simulink subsystem "HMT"  (R2022b)
settings: Solver=VariableStepAuto  StartTime=0.0  StopTime=10.0  RelTol=1e-3
libraries: fl_lib x21, nesl_utility x17, sh_lib x8, sdl_lib x4
settings Model: Creator=david  LastModifiedBy=david

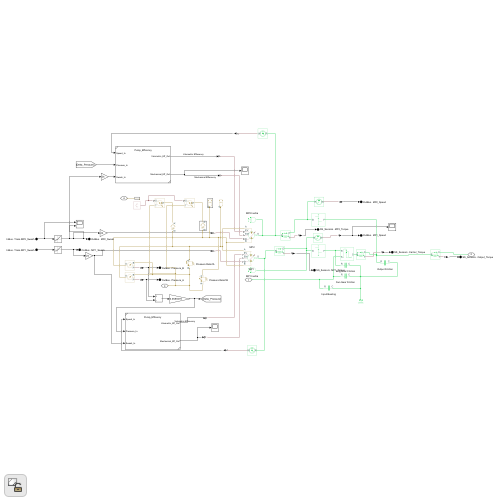
[thumbnail: Simulink's stored preview of the top-level diagram]
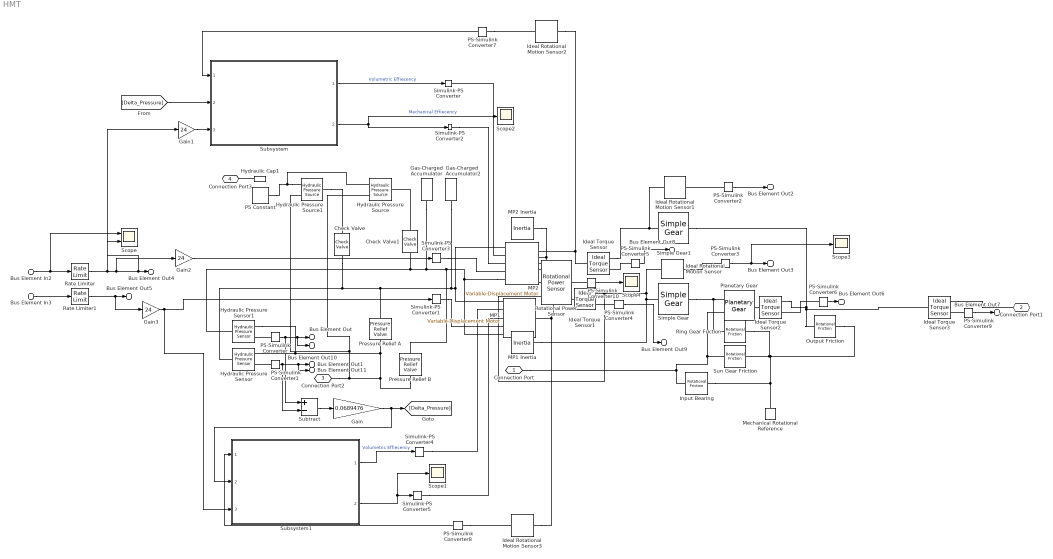
== system HMT ==
  Bus Element In3 : Inport  PortName=InBus  Element=MP1_Swash
  Bus Element In2 : Inport  PortName=InBus  Element=MP2_Swash
  Check Valve : sh_lib/Valves/Directional Valves/Check Valve  area_max=1e-4 m^2  pres_crack=0.3e5 Pa  pres_max=1.2e5 Pa  C_d=0.7  A_leak=.001 in^2  lam_spec=1  B_lam=0.999  Re_cr=12  dynamic=0  tau=0.1 s  area_init=1e-12 m^2
      settings: InternalSimscapePortConfiguration="{\"Bottom\":[],\"Left\":[{\"id\":\"A\",\"label\":\"A\",\"type\":\"foundation.hydraulic.hydraulic\"}],\"Right\":[{\"id\":\"B\",\"label\":\"B\",\"type\":\"foundation.hydraulic.hydraulic\"}],\"Top\":[]}"
  Check Valve1 : sh_lib/Valves/Directional Valves/Check Valve  area_max=1e-4 m^2  pres_crack=0.3e5 Pa  pres_max=1.2e5 Pa  C_d=0.7  A_leak=.001 in^2  lam_spec=1  B_lam=0.999  Re_cr=12  dynamic=0  tau=0.1 s  area_init=1e-12 m^2
      settings: InternalSimscapePortConfiguration="{\"Bottom\":[],\"Left\":[{\"id\":\"A\",\"label\":\"A\",\"type\":\"foundation.hydraulic.hydraulic\"}],\"Right\":[{\"id\":\"B\",\"label\":\"B\",\"type\":\"foundation.hydraulic.hydraulic\"}],\"Top\":[]}"
  Gain : Gain  Gain=0.0689476
  Gain1 : Gain  Gain=24
  Gain2 : Gain  Gain=24
  Gain3 : Gain  Gain=24
  Gas-Charged Accumulator : sh_lib/Accumulators/Gas-Charged Accumulator  capacity=2 in^3  dead_volume=1 in^3  pr_preload=2000 psi  k_sh=1.4  stiff_coeff=1e10 Pa/m^3  penetr_coeff=1e10 Pa*s/m^6  flow_rate_specify=off  flow_rate_priority=None  flow_rate=5e-3 m^3/s  flow_rate_nominal_specify=off  flow_rate_nominal_unit=m^3/s  flow_rate_nominal_value=1  liquid_volume_specify=on  liquid_volume_priority=High  liquid_volume=1 in^3  liquid_volume_nominal_specify=off  liquid_volume_nominal_unit=m^3  liquid_volume_nominal_value=1  liquid_pressure_specify=off  liquid_pressure_priority=None  liquid_pressure=1.01325e5 Pa  liquid_pressure_nominal_specify=off  liquid_pressure_nominal_unit=Pa  liquid_pressure_nominal_value=1
      settings: InternalSimscapePortConfiguration="{\"Bottom\":[],\"Left\":[],\"Right\":[{\"id\":\"A\",\"label\":\"A\",\"type\":\"foundation.hydraulic.hydraulic\"}],\"Top\":[]}"
  Gas-Charged Accumulator2 : sh_lib/Accumulators/Gas-Charged Accumulator  capacity=2 in^3  dead_volume=1 in^3  pr_preload=2000 psi  k_sh=1.4  stiff_coeff=1e10 Pa/m^3  penetr_coeff=1e10 Pa*s/m^6  flow_rate_specify=off  flow_rate_priority=None  flow_rate=5e-3 m^3/s  flow_rate_nominal_specify=off  flow_rate_nominal_unit=m^3/s  flow_rate_nominal_value=1  liquid_volume_specify=on  liquid_volume_priority=High  liquid_volume=1 in^3  liquid_volume_nominal_specify=off  liquid_volume_nominal_unit=m^3  liquid_volume_nominal_value=1  liquid_pressure_specify=off  liquid_pressure_priority=None  liquid_pressure=1.01325e5 Pa  liquid_pressure_nominal_specify=off  liquid_pressure_nominal_unit=Pa  liquid_pressure_nominal_value=1
      settings: InternalSimscapePortConfiguration="{\"Bottom\":[],\"Left\":[],\"Right\":[{\"id\":\"A\",\"label\":\"A\",\"type\":\"foundation.hydraulic.hydraulic\"}],\"Top\":[]}"
  Hydraulic Cap1 : fl_lib/Hydraulic/Hydraulic Elements/Hydraulic Cap  p_specify=off  p_priority=None  p=0 Pa  p_nominal_specify=off  p_nominal_unit=Pa  p_nominal_value=1
      settings: InternalSimscapePortConfiguration="{\"Bottom\":[],\"Left\":[{\"id\":\"P\",\"label\":\"\",\"type\":\"foundation.hydraulic.hydraulic\"}],\"Right\":[],\"Top\":[]}"
  Hydraulic Pressure Sensor : fl_lib/Hydraulic/Hydraulic Sensors/Hydraulic Pressure Sensor
  Hydraulic Pressure Sensor1 : fl_lib/Hydraulic/Hydraulic Sensors/Hydraulic Pressure Sensor
  Hydraulic Pressure Source : fl_lib/Hydraulic/Hydraulic Sources/Hydraulic Pressure Source
      settings: InternalSimscapePortConfiguration="{\"Bottom\":[],\"Left\":[{\"id\":\"P\",\"label\":\"P\",\"type\":\"foundation.hydraulic.hydraulic\"}],\"Right\":[{\"id\":\"S\",\"label\":\"S\",\"type\":\"input\"},{\"id\":\"T\",\"label\":\"T\",\"type\":\"foundation.hydraulic.hydraulic\"}],\"Top\":[]}"
  Hydraulic Pressure Source1 : fl_lib/Hydraulic/Hydraulic Sources/Hydraulic Pressure Source
      settings: InternalSimscapePortConfiguration="{\"Bottom\":[],\"Left\":[{\"id\":\"P\",\"label\":\"P\",\"type\":\"foundation.hydraulic.hydraulic\"}],\"Right\":[{\"id\":\"S\",\"label\":\"S\",\"type\":\"input\"},{\"id\":\"T\",\"label\":\"T\",\"type\":\"foundation.hydraulic.hydraulic\"}],\"Top\":[]}"
  Ideal Rotational Motion Sensor{,1..3} (4 alike) : fl_lib/Mechanical/Mechanical Sensors/Ideal Rotational Motion Sensor  reference=foundation.enum.MeasurementReference.absolute  acceleration_port=false  velocity_port=true  position_port=false  wrap_angle=false  offset=0 rad
      settings: InternalSimscapePortConfiguration="{\"Bottom\":[],\"Left\":[{\"id\":\"R\",\"label\":\"R\",\"type\":\"foundation.mechanical.rotational.rotational\"}],\"Right\":[{\"id\":\"W\",\"label\":\"W\",\"type\":\"output\"}],\"Top\":[]}"
  Ideal Torque Sensor{,1..3} (4 alike) : fl_lib/Mechanical/Mechanical Sensors/Ideal Torque Sensor
  Input Bearing : fl_lib/Mechanical/Rotational Elements/Rotational Friction  brkwy_trq=1 lbf*ft  brkwy_vel=0.1 rad/s  Col_trq=.5 lbf*ft  visc_coef=0.001 N*m*s/rad  w_specify=off  w_priority=None  w=0 rad/s  w_nominal_specify=off  w_nominal_unit=rad/s  w_nominal_value=1  t_specify=off  t_priority=None  t=0 N*m  t_nominal_specify=off  t_nominal_unit=N*m  t_nominal_value=1
  MP1 : sh_lib/Pumps and Motors/Variable-Displacement Motor  mdl_type=2  stroke_max=1 m  D_max=24 cm^3/rev  cntrl_mem_tab=[-1,0,1] m  displ_tab=[-24,0,24] cm^3/rev  interp_method=2  extrap_method=2  loss_spec=1  w_nominal=4000 rpm  pr_nominal=2000 psi  visc_nominal=18 cSt  dens_nominal=900 kg/m^3  efficiency_vol=0.95  no_load_torque=0.05 N*m  torque_pressure_coeff=0.6e-6 N*m/Pa  p_diff_eff_TLU=[10,135,278] bar  omega_eff_TLU=[500,1974,4000] rpm  displacement_eff_TLU=[4.8,12,24] cm^3/rev  vol_eff_TLU=cat(3,[.47,0.01,0.01; .98,.38,.01;.98,.67,.38],[.81,.12,0.01;.99,.80,.65;1.00,.88,.79],[.93,.61,.42;1.00,.91,.85;1.00,.95,.89])  mech_eff_TLU=cat(3,[.46,.62,.54;.27,.74,.83;.21,.73,.89],[.65,.86,.83;.46,.86,.94;.35,.86,.95],[.66,.83,.85;.53,.88,.91;.39,.87,.94])  p_diff_loss_TLU=[100000, 1000000, 2000000] Pa  omega_loss_TLU=[25, 50, 100, 200, 300, 400] rad/s  displacement_loss_TLU=[-30, -19, 19, 30] cm^3/rev  vol_loss_TLU=repmat([.0282, .0253, .0241, .0235, .0291, .0325; .2596, .1271, .1017, .0917, .1216, .1142; .7874, .1901, .141, .1211, .1797, .1978] * 1e-3, 1, 1, 4) m^3/s  mech_loss_TLU=repmat([.002, .002, .002, .002, .002, .002; .06, .055, .055, .055, .055, .05; .19, .19, .18, .18, .17, .16], 1, 1, 4) N*m  pressure_threshold=10 psi  omega_threshold=10 rad/s  displacement_threshold=0.5 cm^3/rev  octant_check=0  pressure_check=0  min_valid_pressure=0 Pa  vol_eff_min=1  vol_eff_max=1  mech_eff_min=.01  mech_eff_max=1
      settings: InternalSimscapePortConfiguration="{\"Bottom\":[],\"Left\":[{\"id\":\"A\",\"label\":\"A\",\"type\":\"foundation.hydraulic.hydraulic\"},{\"id\":\"EV\",\"label\":\"EV\",\"type\":\"input\"},{\"id\":\"EM\",\"label\":\"EM\",\"type\":\"input\"},{\"id\":\"D\",\"label\":\"D\",\"type\":\"input\"},{\"id\":\"B\",\"label\":\"B\",\"type\":\"foundation.hydraulic.hydraulic\"}],\"Right\":[{\"id\":\"S\",\"label\":\"S\",\"type\":\"foundation.mechanical.rotational.rotational\"}],\"Top\":[]}"
  MP1 Inertia : fl_lib/Mechanical/Rotational Elements/Inertia  inertia=0.0009 kg*m^2  num_ports=foundation.enum.numPorts2.one  w_specify=off  w_priority=Low  w=0 rad/s  w_nominal_specify=off  w_nominal_unit=rad/s  w_nominal_value=1  t_specify=off  t_priority=None  t=0 N*m  t_nominal_specify=off  t_nominal_unit=N*m  t_nominal_value=1
  MP2 : sh_lib/Pumps and Motors/Variable-Displacement Motor  mdl_type=2  stroke_max=1 m  D_max=24 cm^3/rev  cntrl_mem_tab=[-1,0,1] m  displ_tab=[-24,0,24] cm^3/rev  interp_method=2  extrap_method=2  loss_spec=1  w_nominal=4000 rpm  pr_nominal=2000 psi  visc_nominal=18 cSt  dens_nominal=900 kg/m^3  efficiency_vol=0.95  no_load_torque=0.05 N*m  torque_pressure_coeff=0.6e-6 N*m/Pa  p_diff_eff_TLU=[10,135,278] bar  omega_eff_TLU=[500,1974,4000] rpm  displacement_eff_TLU=[4.8,12,24] cm^3/rev  vol_eff_TLU=cat(3,[.47,0.01,0.01; .98,.38,.01;.98,.67,.38],[.81,.12,0.01;.99,.80,.65;1.00,.88,.79],[.93,.61,.42;1.00,.91,.85;1.00,.95,.89])  mech_eff_TLU=cat(3,[.46,.62,.54;.27,.74,.83;.21,.73,.89],[.65,.86,.83;.46,.86,.94;.35,.86,.95],[.66,.83,.85;.53,.88,.91;.39,.87,.94])  p_diff_loss_TLU=[100000, 1000000, 2000000] Pa  omega_loss_TLU=[25, 50, 100, 200, 300, 400] rad/s  displacement_loss_TLU=[-30, -19, 19, 30] cm^3/rev  vol_loss_TLU=repmat([.0282, .0253, .0241, .0235, .0291, .0325; .2596, .1271, .1017, .0917, .1216, .1142; .7874, .1901, .141, .1211, .1797, .1978] * 1e-3, 1, 1, 4) m^3/s  mech_loss_TLU=repmat([.002, .002, .002, .002, .002, .002; .06, .055, .055, .055, .055, .05; .19, .19, .18, .18, .17, .16], 1, 1, 4) N*m  pressure_threshold=10 psi  omega_threshold=10 rad/s  displacement_threshold=0.5 cm^3/rev  octant_check=0  pressure_check=0  min_valid_pressure=0 Pa  vol_eff_min=.01  vol_eff_max=1  mech_eff_min=.01  mech_eff_max=1
      settings: InternalSimscapePortConfiguration="{\"Bottom\":[],\"Left\":[{\"id\":\"A\",\"label\":\"A\",\"type\":\"foundation.hydraulic.hydraulic\"},{\"id\":\"EV\",\"label\":\"EV\",\"type\":\"input\"},{\"id\":\"EM\",\"label\":\"EM\",\"type\":\"input\"},{\"id\":\"D\",\"label\":\"D\",\"type\":\"input\"},{\"id\":\"B\",\"label\":\"B\",\"type\":\"foundation.hydraulic.hydraulic\"}],\"Right\":[{\"id\":\"S\",\"label\":\"S\",\"type\":\"foundation.mechanical.rotational.rotational\"}],\"Top\":[]}"
  MP2 Inertia : fl_lib/Mechanical/Rotational Elements/Inertia  inertia=0.0009 kg*m^2  num_ports=foundation.enum.numPorts2.one  w_specify=on  w_priority=Low  w=0 rpm  w_nominal_specify=off  w_nominal_unit=rad/s  w_nominal_value=1  t_specify=off  t_priority=None  t=0 N*m  t_nominal_specify=off  t_nominal_unit=N*m  t_nominal_value=1
  Mechanical Rotational Reference : fl_lib/Mechanical/Rotational Elements/Mechanical Rotational Reference
  Output Friction : fl_lib/Mechanical/Rotational Elements/Rotational Friction  brkwy_trq=1 lbf*ft  brkwy_vel=0.1 rad/s  Col_trq=.5 lbf*ft  visc_coef=0.001 N*m*s/rad  w_specify=off  w_priority=None  w=0 rad/s  w_nominal_specify=off  w_nominal_unit=rad/s  w_nominal_value=1  t_specify=off  t_priority=None  t=0 N*m  t_nominal_specify=off  t_nominal_unit=N*m  t_nominal_value=1
  PS Constant : fl_lib/Physical Signals/Sources/PS Constant  constant=100 psi
  PS-Simulink Converter : nesl_utility/PS-Simulink Converter  PhysicalDomain=network_engine_domain  SubClassName=ps_output  LeftPortType=input  RightPortType=output  PseudoPeriodic=off  Frequencies=[]  VectorFormat=inherit  Unit=psi  AffineConversion=off
  PS-Simulink Converter1 : nesl_utility/PS-Simulink Converter  PhysicalDomain=network_engine_domain  SubClassName=ps_output  LeftPortType=input  RightPortType=output  PseudoPeriodic=off  Frequencies=[]  VectorFormat=inherit  Unit=psi  AffineConversion=off
  PS-Simulink Converter10 : nesl_utility/PS-Simulink Converter  PhysicalDomain=network_engine_domain  SubClassName=ps_output  LeftPortType=input  RightPortType=output  PseudoPeriodic=off  Frequencies=[]  VectorFormat=inherit  Unit=inherit  AffineConversion=off
  PS-Simulink Converter{2..3,7..8} (4 alike) : nesl_utility/PS-Simulink Converter  PhysicalDomain=network_engine_domain  SubClassName=ps_output  LeftPortType=input  RightPortType=output  PseudoPeriodic=off  Frequencies=[]  VectorFormat=inherit  Unit=rpm  AffineConversion=off
  PS-Simulink Converter4 : nesl_utility/PS-Simulink Converter  PhysicalDomain=network_engine_domain  SubClassName=ps_output  LeftPortType=input  RightPortType=output  PseudoPeriodic=off  Frequencies=[]  VectorFormat=inherit  Unit=in*lb  AffineConversion=off
  PS-Simulink Converter5 : nesl_utility/PS-Simulink Converter  PhysicalDomain=network_engine_domain  SubClassName=ps_output  LeftPortType=input  RightPortType=output  PseudoPeriodic=off  Frequencies=[]  VectorFormat=inherit  Unit=in*lb  AffineConversion=off
  PS-Simulink Converter6 : nesl_utility/PS-Simulink Converter  PhysicalDomain=network_engine_domain  SubClassName=ps_output  LeftPortType=input  RightPortType=output  PseudoPeriodic=off  Frequencies=[]  VectorFormat=inherit  Unit=ft*lb  AffineConversion=off
  PS-Simulink Converter9 : nesl_utility/PS-Simulink Converter  PhysicalDomain=network_engine_domain  SubClassName=ps_output  LeftPortType=input  RightPortType=output  PseudoPeriodic=off  Frequencies=[]  VectorFormat=inherit  Unit=ft*lb  AffineConversion=off
  Planetary Gear : sdl_lib/Gears/Planetary Gear  rs_ratio=2.636  friction_model=sdl.enum.gear_friction.constant  efficiency=[.96, .98]  temperature_TLU=[280, 300, 320] K  efficiency_sp_TLU=[.95, .9, .85]  efficiency_rp_TLU=[.95, .9, .85]  pwr_thr=[.001, .001] W  mu_visc=[0, 0] N*m*s/rad  model_inertia=simscape.enum.onoff.off  planet_inertia=0.001 kg*m^2  thermal_mass=50 J/K  T_init=300 K
  Pressure Relief A : sh_lib/Valves/Pressure Control Valves/Pressure Relief Valve  valve_area_spec=1  p_diff_TLU=[30.15e5 : 15e3 : 31.35e5] Pa  area_TLU=[1 : 1 : 9] .* 1e-5 m^2  area_max=1e-4 m^2  pres_set=4000 psi  reg_range=5e5 Pa  C_d=0.7  A_leak=1e-12 m^2  lam_spec=1  B_lam=0.999  Re_cr=12  dynamic=0  tau=0.1 s  area_init=1e-12 m^2
      settings: InternalSimscapePortConfiguration="{\"Bottom\":[],\"Left\":[{\"id\":\"A\",\"label\":\"A\",\"type\":\"foundation.hydraulic.hydraulic\"}],\"Right\":[{\"id\":\"B\",\"label\":\"B\",\"type\":\"foundation.hydraulic.hydraulic\"}],\"Top\":[]}"
  Pressure Relief B : sh_lib/Valves/Pressure Control Valves/Pressure Relief Valve  valve_area_spec=1  p_diff_TLU=[30.15e5 : 15e3 : 31.35e5] Pa  area_TLU=[1 : 1 : 9] .* 1e-5 m^2  area_max=1e-4 m^2  pres_set=4000 psi  reg_range=5e5 Pa  C_d=0.7  A_leak=1e-12 m^2  lam_spec=1  B_lam=0.999  Re_cr=12  dynamic=0  tau=0.1 s  area_init=1e-12 m^2
      settings: InternalSimscapePortConfiguration="{\"Bottom\":[],\"Left\":[{\"id\":\"A\",\"label\":\"A\",\"type\":\"foundation.hydraulic.hydraulic\"}],\"Right\":[{\"id\":\"B\",\"label\":\"B\",\"type\":\"foundation.hydraulic.hydraulic\"}],\"Top\":[]}"
  Rate Limiter : RateLimiter  RisingSlewLimit=.5  FallingSlewLimit=-.5  SampleTimeMode=inherited
  Rate Limiter1 : RateLimiter  RisingSlewLimit=.5  FallingSlewLimit=-.5  SampleTimeMode=inherited
  Ring Gear Friction : fl_lib/Mechanical/Rotational Elements/Rotational Friction  brkwy_trq=1 lbf*ft  brkwy_vel=0.1 rad/s  Col_trq=.5 lbf*ft  visc_coef=0.001 N*m*s/rad  w_specify=off  w_priority=None  w=0 rad/s  w_nominal_specify=off  w_nominal_unit=rad/s  w_nominal_value=1  t_specify=off  t_priority=None  t=0 N*m  t_nominal_specify=off  t_nominal_unit=N*m  t_nominal_value=1
  Rotational Power Sensor : sdl_lib/Sensors/Rotational Power Sensor  measurement_type=sdl.enum.rotationalPowerSensorType.instantaneous  averaging_period=1 s  max_frequency=1000 Hz  max_speed=1000 rpm
      settings: InternalSimscapePortConfiguration="{\"Bottom\":[],\"Left\":[{\"id\":\"S\",\"label\":\"S\",\"type\":\"foundation.mechanical.rotational.rotational\"},{\"id\":\"R\",\"label\":\"R\",\"type\":\"foundation.mechanical.rotational.rotational\"},{\"id\":\"C\",\"label\":\"C\",\"type\":\"foundation.mechanical.rotational.rotational\"}],\"Right\":[{\"id\":\"P\",\"label\":\"P\",\"type\":\"output\"}],\"Top\":[]}"
  Scope : Scope  NumInputPorts=2
  Scope{1..4} (4 alike) : Scope
  Simple Gear : sdl_lib/Gears/Simple Gear  ratio=2.16  rotation_direction=sdl.enum.shaftOutputDirection.opposite  friction_model=sdl.enum.gear_efficiencies_load.constant  T_noload=0.1 N*m  T_nom=5 N*m  efficiency_nom=0.8  efficiency=0.98  temperature_TLU=[280, 300, 320] K  load_TLU=[1, 5, 10] N*m  efficiency_TLU=[.95, .9, .85]  efficiency_TLU2=[.85, .8, .75; .95, .9, .85; .85, .8, .7]  w_thr=0.01 rad/s  pwr_thr=0.001 W  backlash_model=sdl.enum.backlashModel.Off  backlash_distance=1e-3 mm  x0=0 mm  r_base=0.1 m  hardstop_model=simscape.enum.hardstop.smooth  transition=1e-4 mm  backlash_stiffness=1e7 N/m  backlash_damping=1e6 N*s/m  e=0  v_tol=0.001 m/s  mu_visc=[0, 0] N*m*s/rad  enable_faults=simscape.enum.onoff.off  efficiency_fault=0.05  external_fault=simscape.enum.onoff.off  temporal_fault=simscape.enum.onoff.off  fault_time=5 s  fault_angles=pi / 12 rad  report_fault=simscape.enum.assert.action.none  thermal_mass=50 J/K  temperature_specify=off  temperature_priority=High  temperature=300 K  temperature_nominal_specify=off  temperature_nominal_unit=K  temperature_nominal_value=1  x_backlash_specify=off  x_backlash_priority=None  x_backlash=0 mm  x_backlash_nominal_specify=off  x_backlash_nominal_unit=mm  x_backlash_nominal_value=1  f_hardstop_specify=off  f_hardstop_priority=None  f_hardstop=0 N  f_hardstop_nominal_specify=off  f_hardstop_nominal_unit=N  f_hardstop_nominal_value=1  v_backlash_specify=off  v_backlash_priority=None  v_backlash=0 m/s  v_backlash_nominal_specify=off  v_backlash_nominal_unit=m/s  v_backlash_nominal_value=1
  Simple Gear1 : sdl_lib/Gears/Simple Gear  ratio=2.714  rotation_direction=sdl.enum.shaftOutputDirection.opposite  friction_model=sdl.enum.gear_efficiencies_load.constant  T_noload=0.1 N*m  T_nom=5 N*m  efficiency_nom=0.8  efficiency=0.98  temperature_TLU=[280, 300, 320] K  load_TLU=[1, 5, 10] N*m  efficiency_TLU=[.95, .9, .85]  efficiency_TLU2=[.85, .8, .75; .95, .9, .85; .85, .8, .7]  w_thr=0.01 rad/s  pwr_thr=0.001 W  backlash_model=sdl.enum.backlashModel.Off  backlash_distance=1e-3 mm  x0=0 mm  r_base=0.1 m  hardstop_model=simscape.enum.hardstop.smooth  transition=1e-4 mm  backlash_stiffness=1e7 N/m  backlash_damping=1e6 N*s/m  e=0  v_tol=0.001 m/s  mu_visc=[0, 0] N*m*s/rad  enable_faults=simscape.enum.onoff.off  efficiency_fault=0.05  external_fault=simscape.enum.onoff.off  temporal_fault=simscape.enum.onoff.off  fault_time=5 s  fault_angles=pi / 12 rad  report_fault=simscape.enum.assert.action.none  thermal_mass=50 J/K  temperature_specify=off  temperature_priority=High  temperature=300 K  temperature_nominal_specify=off  temperature_nominal_unit=K  temperature_nominal_value=1  x_backlash_specify=off  x_backlash_priority=None  x_backlash=0 mm  x_backlash_nominal_specify=off  x_backlash_nominal_unit=mm  x_backlash_nominal_value=1  f_hardstop_specify=off  f_hardstop_priority=None  f_hardstop=0 N  f_hardstop_nominal_specify=off  f_hardstop_nominal_unit=N  f_hardstop_nominal_value=1  v_backlash_specify=off  v_backlash_priority=None  v_backlash=0 m/s  v_backlash_nominal_specify=off  v_backlash_nominal_unit=m/s  v_backlash_nominal_value=1
  Simulink-PS Converter{,2,4..5} (4 alike) : nesl_utility/Simulink-PS Converter  PhysicalDomain=network_engine_domain  SubClassName=ps_input  LeftPortType=input  RightPortType=output  PseudoPeriodic=off  Frequencies=[]  NoiseDistribution=none  NoiseParameters=[]  Unit=1  AffineConversion=off  FilteringAndDerivatives=provide  SimscapeFilterOrder=1  InputFilterTimeConstant=0.001  UdotUserProvided=0
  Simulink-PS Converter1 : nesl_utility/Simulink-PS Converter  PhysicalDomain=network_engine_domain  SubClassName=ps_input  LeftPortType=input  RightPortType=output  PseudoPeriodic=off  Frequencies=[]  NoiseDistribution=none  NoiseParameters=[]  Unit=cm^3/rev  AffineConversion=off  FilteringAndDerivatives=provide  SimscapeFilterOrder=1  InputFilterTimeConstant=0.001  UdotUserProvided=0
  Simulink-PS Converter3 : nesl_utility/Simulink-PS Converter  PhysicalDomain=network_engine_domain  SubClassName=ps_input  LeftPortType=input  RightPortType=output  PseudoPeriodic=off  Frequencies=[]  NoiseDistribution=none  NoiseParameters=[]  Unit=cm^3/rev  AffineConversion=off  FilteringAndDerivatives=provide  SimscapeFilterOrder=1  InputFilterTimeConstant=0.001  UdotUserProvided=0
  Subsystem : Subsystem  ReferencedSubsystem=Pump_Efficency
  Subsystem1 : Subsystem  ReferencedSubsystem=Pump_Efficency
  Subtract : Sum  Inputs=+-
  Sun Gear Friction : fl_lib/Mechanical/Rotational Elements/Rotational Friction  brkwy_trq=1 lbf*ft  brkwy_vel=0.1 rad/s  Col_trq=.5 lbf*ft  visc_coef=0.001 N*m*s/rad  w_specify=off  w_priority=None  w=0 rad/s  w_nominal_specify=off  w_nominal_unit=rad/s  w_nominal_value=1  t_specify=off  t_priority=None  t=0 N*m  t_nominal_specify=off  t_nominal_unit=N*m  t_nominal_value=1
  Connection Port : PMIOPort  Side=Right
  Connection Port1 : PMIOPort  Port=2  Side=Left
  Connection Port2 : PMIOPort  Port=3  Side=Right
  Connection Port3 : PMIOPort  Port=4  Side=Left
  Bus Element Out : Outport  VectorParamsAs1DForOutWhenUnconnected=off  PortName=OutBus  Element=Pressure_B
  Bus Element Out1 : Outport  VectorParamsAs1DForOutWhenUnconnected=off  PortName=OutBus  Element=Pressure_A
  Bus Element Out2 : Outport  VectorParamsAs1DForOutWhenUnconnected=off  PortName=OutBus  Element=MP2_Speed
  Bus Element Out3 : Outport  VectorParamsAs1DForOutWhenUnconnected=off  PortName=OutBus  Element=MP1_Speed
  Bus Element Out4 : Outport  VectorParamsAs1DForOutWhenUnconnected=off  PortName=OutBus  Element=MP2_Swash
  Bus Element Out5 : Outport  VectorParamsAs1DForOutWhenUnconnected=off  PortName=OutBus  Element=MP1_Swash
  Bus Element Out9 : Outport  Port=2  VectorParamsAs1DForOutWhenUnconnected=off  PortName=SS_Sensors  Element=MP1_Torque
  Bus Element Out8 : Outport  Port=2  VectorParamsAs1DForOutWhenUnconnected=off  PortName=SS_Sensors  Element=MP2_Torque
  Bus Element Out6 : Outport  Port=2  VectorParamsAs1DForOutWhenUnconnected=off  PortName=SS_Sensors  Element=Carrier_Torque
  Bus Element Out7 : Outport  Port=2  VectorParamsAs1DForOutWhenUnconnected=off  PortName=SS_Sensors  Element=Output_Torque
  Bus Element Out10 : Outport  Port=2  VectorParamsAs1DForOutWhenUnconnected=off  PortName=SS_Sensors  Element=Pressure_B
  Bus Element Out11 : Outport  Port=2  VectorParamsAs1DForOutWhenUnconnected=off  PortName=SS_Sensors  Element=Pressure_A
  wires:
  PS-Simulink Converter10/1 -> Scope4/1
  PS-Simulink Converter9/1 -> Bus Element Out7/1
  Gain1/1 -> Subsystem/3
  PS-Simulink Converter7/1 -> Subsystem/1
  Bus Element In2/1 -> Rate Limiter/1, Scope/1
  Rate Limiter1/1 -> Gain3/1, Bus Element Out5/1
  Bus Element In3/1 -> Rate Limiter1/1
  PS-Simulink Converter3/1 -> Bus Element Out3/1, Scope3/1
  PS-Simulink Converter2/1 -> Bus Element Out2/1
  PS-Simulink Converter/1 -> Bus Element Out/1, Bus Element Out10/1, Subtract/1
  PS-Simulink Converter1/1 -> Bus Element Out1/1, Bus Element Out11/1, Subtract/2
  PS-Simulink Converter5/1 -> Bus Element Out8/1
  PS-Simulink Converter6/1 -> Bus Element Out6/1
  PS-Simulink Converter4/1 -> Bus Element Out9/1
  Subsystem/1 -> Simulink-PS Converter/1  "Volumetric Effiecency"
  Subsystem/2 -> Simulink-PS Converter2/1, Scope2/1  "Mechanical Effiecency"
  Subtract/1 -> Gain/1
  [Delta_Pressure] -> Subsystem/2
  Rate Limiter/1 -> Scope/2, Gain2/1, Gain1/1, Bus Element Out4/1
  Gain2/1 -> Simulink-PS Converter3/1
  Subsystem1/1 -> Simulink-PS Converter4/1  "Volumetric Effiecency"
  PS-Simulink Converter8/1 -> Subsystem1/1
  Gain3/1 -> Subsystem1/3, Simulink-PS Converter1/1
  Gain/1 -> Subsystem1/2, [Delta_Pressure]
  Subsystem1/2 -> Simulink-PS Converter5/1, Scope1/1
  connections:
  Rotational Power Sensor/LConn2 -- Ideal Rotational Motion Sensor2/LConn1 -- Ideal Torque Sensor/LConn1
  Input Bearing/RConn1 -- Ring Gear Friction/RConn1 -- Sun Gear Friction/RConn1 -- Output Friction/RConn1 -- Mechanical Rotational Reference/LConn1
  Planetary Gear/RConn1 -- Ring Gear Friction/LConn1 -- Simple Gear/RConn1
  Sun Gear Friction/LConn1 -- Connection Port/RConn1 -- Input Bearing/LConn1 -- Planetary Gear/RConn2
  Hydraulic Pressure Source1/RConn1 -- Hydraulic Pressure Source/RConn1 -- PS Constant/RConn1
  MP2/LConn5 -- Hydraulic Pressure Sensor1/LConn1 -- Check Valve1/RConn1 -- Gas-Charged Accumulator/RConn1 -- Pressure Relief B/LConn1 -- MP1/LConn5
  MP2/RConn1 -- MP2 Inertia/LConn1 -- Rotational Power Sensor/LConn1
  Ideal Torque Sensor1/RConn1 -- MP1 Inertia/LConn1 -- Simple Gear/LConn1 -- Ideal Rotational Motion Sensor/LConn1 -- Rotational Power Sensor/LConn3
  Output Friction/LConn1 -- Ideal Torque Sensor2/RConn1 -- Simple Gear1/RConn1 -- Ideal Torque Sensor3/LConn1
  Hydraulic Pressure Source1/RConn2 -- Hydraulic Pressure Sensor/RConn1 -- Hydraulic Pressure Sensor1/RConn1 -- Pressure Relief A/RConn1 -- Pressure Relief B/RConn1 -- Connection Port2/RConn1 -- Hydraulic Pressure Source/RConn2
  Hydraulic Pressure Sensor/LConn1 -- MP2/LConn1 -- MP1/LConn1 -- Gas-Charged Accumulator2/RConn1 -- Pressure Relief A/LConn1 -- Check Valve/RConn1
  Ideal Torque Sensor/RConn1 -- Simple Gear1/LConn1 -- Ideal Rotational Motion Sensor1/LConn1
  Ideal Rotational Motion Sensor3/LConn1 -- MP1/RConn1 -- Ideal Torque Sensor1/LConn1
  PS-Simulink Converter10/LConn1 -- Rotational Power Sensor/RConn1
  PS-Simulink Converter9/LConn1 -- Ideal Torque Sensor3/RConn2
  Ideal Torque Sensor3/RConn1 -- Connection Port1/RConn1
  Check Valve1/LConn1 -- Hydraulic Pressure Source/LConn1
  Hydraulic Pressure Source1/LConn1 -- Check Valve/LConn1
  Hydraulic Cap1/LConn1 -- Connection Port3/RConn1
  PS-Simulink Converter3/LConn1 -- Ideal Rotational Motion Sensor/RConn1
  PS-Simulink Converter2/LConn1 -- Ideal Rotational Motion Sensor1/RConn1
  PS-Simulink Converter1/LConn1 -- Hydraulic Pressure Sensor/RConn2
  PS-Simulink Converter/LConn1 -- Hydraulic Pressure Sensor1/RConn2
  PS-Simulink Converter4/LConn1 -- Ideal Torque Sensor1/RConn2
  PS-Simulink Converter5/LConn1 -- Ideal Torque Sensor/RConn2
  Ideal Torque Sensor2/LConn1 -- Planetary Gear/LConn1
  PS-Simulink Converter6/LConn1 -- Ideal Torque Sensor2/RConn2
  Simulink-PS Converter3/RConn1 -- MP2/LConn4
  Simulink-PS Converter2/RConn1 -- MP2/LConn3
  MP2/LConn2 -- Simulink-PS Converter/RConn1
  PS-Simulink Converter7/LConn1 -- Ideal Rotational Motion Sensor2/RConn1
  Simulink-PS Converter4/RConn1 -- MP1/LConn2
  Simulink-PS Converter5/RConn1 -- MP1/LConn3
  Simulink-PS Converter1/RConn1 -- MP1/LConn4
  PS-Simulink Converter8/LConn1 -- Ideal Rotational Motion Sensor3/RConn1
